simulink model "sl_fforward"  (R2016a)
settings: Solver=ode45  StartTime=0.0  StopTime=10.0  RelTol=1e-3
values from neighbouring files (symbols this model uses):
  p560 = p560.nofriction    [problem_1.m]    (also in problem_2a.m; problem_2b.m = p560.perturb(0.15); problem_4.m)
libraries: roblocks x4
settings Model: Creator=corkep  LastModifiedBy=magiccjae
settings DataIOCC: LimitDataPoints=on  SaveFormat=Array  SignalLoggingSaveFormat=ModelDataLogs
settings OptimizationCC: ExpressionDepthLimit=2147483647
settings DebuggingCC: UnderspecifiedInitializationDetection=Classic  MergeDetectMultiDrivingBlocksExec=none  SolverPrmCheckMsg=warning  FcnCallInpInsideContextMsg=UseLocalSettings  StateNameClashWarn=warning
settings HardwareCC: ProdBitPerPointer=32  ProdLargestAtomicFloat=None  ProdIntDivRoundTo=Undefined  ProdEndianess=Unspecified  ProdWordSize=32  ProdHWDeviceType=32-bit Generic
settings ModelReferenceCC: PropagateSignalLabelsOutOfModel=off
settings GRTTargetCC: CombineOutputUpdateFcns=off  GRTInterface=on
settings ConfigComp: CovModelRefEnable=Off

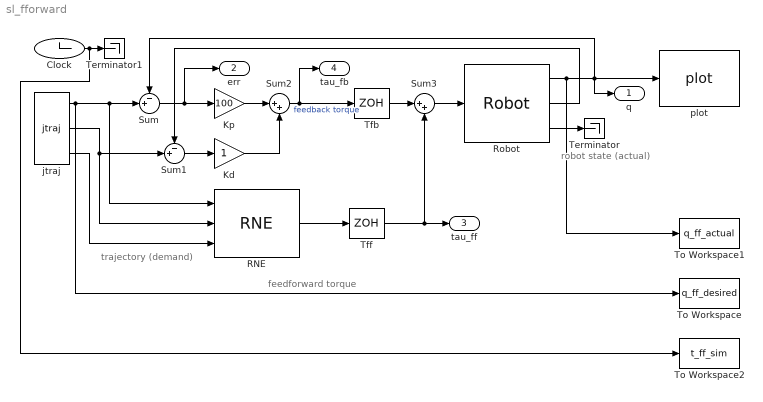
== system sl_fforward ==
  note: trajectory
      | (demand)
  note: robot state
      | (actual)
  note: feedforward torque
  Clock : Clock
  Kd : Gain  SaturateOnIntegerOverflow=on  OutDataTypeStr=Inherit: Same as input  ParamDataTypeStr=Inherit: Same as input
  Kp : Gain  Gain=100  SaturateOnIntegerOverflow=on  OutDataTypeStr=Inherit: Same as input  ParamDataTypeStr=Inherit: Same as input
  RNE : roblocks/Dynamics/RNE  robot=p560.nofriction()  grav=[0 0 9.81]
  Robot : roblocks/Dynamics/Robot  robot=p560  q0=[0 0 0 0 0 0]
  Sum : Sum  Inputs=-+|  SaturateOnIntegerOverflow=on  InputSameDT=on  OutDataTypeStr=Inherit: Same as first input
  Sum1 : Sum  Inputs=-+|  SaturateOnIntegerOverflow=on  InputSameDT=on  OutDataTypeStr=Inherit: Same as first input
  Sum2 : Sum  Inputs=|++  SaturateOnIntegerOverflow=on  InputSameDT=on  OutDataTypeStr=Inherit: Same as first input
  Sum3 : Sum  Inputs=|++  SaturateOnIntegerOverflow=on  InputSameDT=on  OutDataTypeStr=Inherit: Same as first input
  Terminator : Terminator
  Terminator1 : Terminator
  Tfb : ZeroOrderHold  SampleTime=0.01
  Tff : ZeroOrderHold  SampleTime=0.01
  To Workspace : ToWorkspace  VariableName=q_ff_desired  SaveFormat=Timeseries  SampleTime=-1
  To Workspace1 : ToWorkspace  VariableName=q_ff_actual  SaveFormat=Timeseries  SampleTime=-1
  To Workspace2 : ToWorkspace  VariableName=t_ff_sim  SaveFormat=Timeseries  SampleTime=-1
  jtraj : roblocks/Trajectory/jtraj  q0=[0 0 0 0 0 0]  qf=[pi/4 pi/2 -pi/2 0 0 0]  tmax=10  ts=-1
  plot : roblocks/Robot Graphics/plot  robot=p560  fps=1  holdplot=on
  q : Outport
  err : Outport  Port=2
  tau_ff : Outport  Port=3
  tau_fb : Outport  Port=4
  wires:
  Kd/1 -> Sum2/2
  Sum/1 -> Kp/1, err/1
  Kp/1 -> Sum2/1
  Sum1/1 -> Kd/1
  Sum2/1 -> Tfb/1, tau_fb/1  "feedback torque"
  Sum3/1 -> Robot/1
  Robot/1 -> plot/1, Sum/1, q/1, To Workspace1/1
  Robot/2 -> Sum1/1
  jtraj/1 -> RNE/1, Sum/2, To Workspace/1
  jtraj/2 -> Sum1/2, RNE/2
  jtraj/3 -> RNE/3
  Robot/3 -> Terminator/1
  Tff/1 -> Sum3/2, tau_ff/1
  Tfb/1 -> Sum3/1
  RNE/1 -> Tff/1
  Clock/1 -> To Workspace2/1, Terminator1/1
